simulink model "h_3D_sim"  (R2018b)
settings: Solver=FixedStepAuto  StartTime=0.0  StopTime=15  FixedStep=0.01  RelTol=1e-3
StopFcn:
  | %g_surface_plot
settings Model: Creator=p282037  LastModifiedBy=weijia
settings OptimizationCC: LifeSpan=inf
settings DebuggingCC: LibraryContextMissingDiagnostic=none  SFExecutionAtInitializationDiag=none
settings SFSimCC: SimUseLocalCustomCode=off
settings RTWCC: RTWUseLocalCustomCode=off
settings CodeAppCC: StateflowObjectComments=on

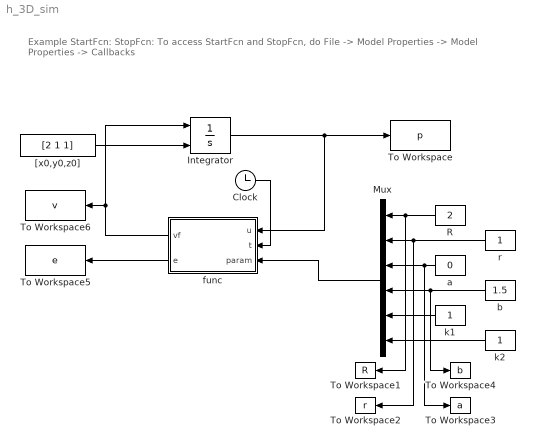
== system h_3D_sim ==
  note: Example
      | StartFcn:
      | StopFcn:
      | To access StartFcn and StopFcn, do File -> Model Properties -> Model Properties -> Callbacks
  Clock : Clock
  Integrator : Integrator  InitialConditionSource=external  InitialCondition=[0 0.5 3]
  Mux : Mux  Inputs=6
  R : Constant  Value=2
  To Workspace : ToWorkspace  VariableName=p  SampleTime=-1
      settings: Save2DSignal=2-D array (concatenate along first dimension)
  To Workspace1 : ToWorkspace  VariableName=R  SampleTime=-1
      settings: MaxDataPoints=1
  To Workspace2 : ToWorkspace  VariableName=r  SampleTime=-1
      settings: MaxDataPoints=1
  To Workspace3 : ToWorkspace  VariableName=a  SampleTime=-1
      settings: MaxDataPoints=1
  To Workspace4 : ToWorkspace  VariableName=b  SampleTime=-1
      settings: MaxDataPoints=1
  To Workspace5 : ToWorkspace  VariableName=e  SaveFormat=Timeseries  SampleTime=-1
  To Workspace6 : ToWorkspace  VariableName=v  SaveFormat=Timeseries  SampleTime=-1
  "[x0,y0,z0]" : Constant  Value=[2 1 1]
  a : Constant  Value=0
  b : Constant  Value=1.5
  func : MATLAB Function  TreatAsAtomicUnit=on
  k1 : Constant
  k2 : Constant
  r : Constant
  wires:
  func/1(vf) -> To Workspace6/1, Integrator/1
  r/1 -> To Workspace2/1, Mux/2
  a/1 -> To Workspace3/1, Mux/3
  b/1 -> To Workspace4/1, Mux/4
  R/1 -> To Workspace1/1, Mux/1
  Mux/1 -> func/3(param)
  "[x0,y0,z0]"/1 -> Integrator/2
  func/2(e) -> To Workspace5/1
  k1/1 -> Mux/5
  k2/1 -> Mux/6
  Integrator/1 -> To Workspace/1, func/1(u)
  Clock/1 -> func/2(t)

== matlab function h_3D_sim/func ==
  data: u input; t input; vf output; param input; e output
function [vf, e] = fcn(u, t, param)

x=u(1); y=u(2); z=u(3);

%%

%%% circle desired path
k11 = 2; k12 = 2;
e11 = x^2 + y^2 - 4;
e12 = z;
n11 = [2*x; 2*y; 0];
n12 = [0; 0; 1];
v1 = cross(n11, n12) - k11*e11*n11 - k12*e12*n12;

%%% sphere reactive area
k2 = 1;
e2 = (x+2)^2 + y^2 +z^2 - 1;
n2 = [2*(x+2); 2*y; 2*z];
% hatn = n2 /norm(n2);
% P = eye(3) - hatn*transpose(hatn);
% a = [0; 0 ;1];
% a = z*[0; 0; 1];
% v2 = P*a - k2*e2*n2;
v2 = cross(n2,[1;0;0]) - k2*e2*n2;

%%%
%% bump fuunctions with different radius mixed vf
c = -0.72;
l1 = 0.1; l2 = 0.1;
if( e2 < c)
    kv1 = 0;
else
    if( e2 < 0 )
        f1 = exp( l1/(c - e2) );
        f2 = exp( l2/(e2 - 0) );
        kv1 = f1/(f1+f2);
    else
        kv1 = 1;
    end
end

kv2 = 1-kv1;

vf = kv1 * v1 / norm(v1) + kv2 * v2 / norm(v2);
e1=sqrt(e11^2+e12^2);
e=[e1; e2];
